simulink model "tether_pull_R2019B"  (R2019b)
settings: Solver=ode4  StartTime=0.0  StopTime=simInit.TSIM  FixedStep=simInit.dt  RelTol=1e-1
InitFcn:
  | close all
undefined symbols (not defined in the file or in its folder): DE2019, ENVMT, simInit, T
libraries: simulink x1, dspmathops x1, dspsigops x1
settings Model: SimulationMode=accelerator  ExtModeTrigDuration=100  Creator=Sebastian  LastModifiedBy=dylaneijkelhof
settings SolverCC: SolverJacobianMethodControl=FullAnalytical
settings DataIOCC: SaveFormat=Array  SaveOutput=off  SignalLogging=off  DSMLogging=off  SaveTime=off  ReturnWorkspaceOutputs=off  StateSaveName=tmp_raccel_xout  SignalLoggingName=logged_signals  LoggingFileName=log
settings OptimizationCC: EfficientMapNaN2IntZero=off
settings DebuggingCC: ArtificialAlgebraicLoopMsg=none  SaveWithDisabledLinksMsg=none  SaveWithParameterizedLinksMsg=none  MaskedZcDiagnostic=none  IgnoredZcDiagnostic=none  InheritedTsInSrcMsg=none  TasksWithSamePriorityMsg=none  SigSpecEnsureSampleTimeMsg=none  ParameterPrecisionLossMsg=none  UnconnectedInputMsg=none  UnconnectedOutputMsg=none  UnconnectedLineMsg=none  BusObjectLabelMismatch=none  RootOutportRequireBusObject=none  AllowSymbolicDim=off  UnknownTsInhSupMsg=none  ModelReferenceDataLoggingMessage=none  ModelReferenceSymbolNameMessage=none  InitInArrayFormatMsg=none  SFUnusedDataAndEventsDiag=none  SFUnexpectedBacktrackingDiag=none  SFInvalidInputDataAccessInChartInitDiag=none  SFNoUnconditionalDefaultTransitionDiag=none  SFTransitionOutsideNaturalParentDiag=none  SFUnreachableExecutionPathDiag=none  SFUndirectedBroadcastEventsDiag=none  SFTransitionActionBeforeConditionDiag=none  SFTemporalDelaySmallerThanSampleTimeDiag=none  SFSelfTransitionDiag=none  SFExecutionAtInitializationDiag=none  SFMachineParentedDataDiag=none  UnitsInconsistencyMsg=none  ArithmeticOperatorsInVariantConditions=warning
settings HardwareCC: ProdBitPerLong=64  ProdHWDeviceType=Intel->x86-64 (Mac OS X)  TargetBitPerLong=64  TargetBitPerPointer=64  TargetBitPerSizeT=64  TargetBitPerPtrDiffT=64  TargetLongLongMode=on  TargetIntDivRoundTo=Zero  TargetEndianess=LittleEndian  TargetWordSize=64  TargetHWDeviceType=MATLAB Host  ProdEqTarget=off
settings ModelReferenceCC: PropagateSignalLabelsOutOfModel=off
settings SFSimCC: SimUseLocalCustomCode=off  CustomCodeUndefinedFunction=UseInterfaceOnly
settings RTWCC: SystemTargetFile=accel.tlc  TemplateMakefile=accel_default_tmf  RTWVerbose=off
settings CodeAppCC: MaxIdLength=128
settings STFCustomTargetCC: TargetLangStandard=C99 (ISO)  ConcurrentExecutionCompliant=on  MATLABClassNameForMDSCustomization=Simulink.SoftwareTarget.TargetSpecificTriggerConfigurationBase  GRTInterface=on  SystemTargetFile=accel.tlc
settings ConfigComp: CovMetricSettings=dw  CovHtmlReporting=on  CovSaveCumulativeToWorkspaceVar=on  CovSaveSingleToWorkspaceVar=on  CovExternalEMLEnable=off

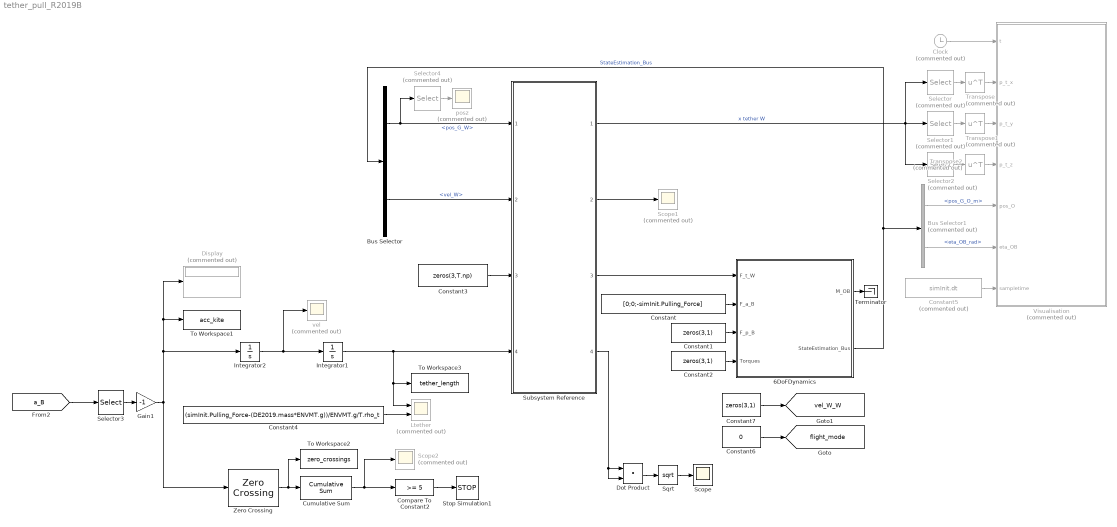
== system tether_pull_R2019B ==
  6DoFDynamics : Subsystem
  Bus Selector : BusSelector  OutputSignals=pos_G_W,vel_W
  Bus Selector1 : BusSelector  Commented=on  OutputSignals=pos_G_O_m,eta_OB_rad
  Clock : Clock  Commented=on
  Compare To Constant2 : simulink/Logic and Bit Operations/Compare To Constant  relop=>=  const=5  OutDataTypeStr=boolean
  Constant : Constant  Value=[0;0;-simInit.Pulling_Force]
  Constant1 : Constant  Value=zeros(3,1)
  Constant2 : Constant  Value=zeros(3,1)
  Constant3 : Constant  Value=zeros(3,T.np)
  Constant4 : Constant  Value=(simInit.Pulling_Force-(DE2019.mass*ENVMT.g))/ENVMT.g/T.rho_t
  Constant5 : Constant  Commented=on  Value=simInit.dt
  Constant6 : Constant  Value=0
  Constant7 : Constant  Value=zeros(3,1)
  Cumulative Sum : dspmathops/Cumulative Sum  dim=Channels (running sum)  InputProcessing=Columns as channels (frame based)  reset_popup=None  roundingMode=Floor  overflowMode=off  outputDataTypeStr=Inherit: Same as accumulator  outputMin=[]  outputMax=[]  outputLastDataTypeStr=Inherit: Same as accumulator
  Display : Display  Commented=on
  Dot Product : DotProduct  InputSameDT=on  OutDataTypeStr=Inherit: Inherit via internal rule
  Gain1 : Gain  Gain=-1
  Integrator1 : Integrator  InitialCondition=T.tether_inital_lenght
  Integrator2 : Integrator
  Ltether : Scope  Commented=on  NumInputPorts=2
  Scope : Scope
  Scope1 : Scope  Commented=on
  Scope2 : Scope  Commented=on
  Selector : Selector  Commented=on  NumberOfDimensions=2  InputPortWidth=3  IndexOptions=Index vector (dialog),Select all  Indices=1,1  OutputSizes=1,1
  Selector1 : Selector  Commented=on  NumberOfDimensions=2  InputPortWidth=3  IndexOptions=Index vector (dialog),Select all  Indices=2,1  OutputSizes=1,1
  Selector2 : Selector  Commented=on  NumberOfDimensions=2  InputPortWidth=3  IndexOptions=Index vector (dialog),Select all  Indices=3,1  OutputSizes=1,1
  Selector3 : Selector  InputPortWidth=3  IndexOptions=Index vector (dialog)  Indices=3  OutputSizes=1
  Selector4 : Selector  Commented=on  InputPortWidth=3  IndexOptions=Index vector (dialog)  Indices=3  OutputSizes=1
  Sqrt : Sqrt  SaturateOnIntegerOverflow=on
  Stop Simulation1 : Stop
  Subsystem Reference : Subsystem  ReferencedSubsystem=Tether_dynamics_R2019B
  Terminator : Terminator
  To Workspace1 : ToWorkspace  VariableName=acc_kite  SaveFormat=Timeseries  SampleTime=-1
  To Workspace2 : ToWorkspace  VariableName=zero_crossings  SaveFormat=Timeseries  SampleTime=-1
  To Workspace3 : ToWorkspace  VariableName=tether_length  SaveFormat=Timeseries  SampleTime=-1
  Transpose : Math  Commented=on  Operator=transpose  SignedPower=off  SaturateOnIntegerOverflow=on
  Transpose1 : Math  Commented=on  Operator=transpose  SignedPower=off  SaturateOnIntegerOverflow=on
  Transpose2 : Math  Commented=on  Operator=transpose  SignedPower=off  SaturateOnIntegerOverflow=on
  Visualisation : MATLAB Function  Commented=on  TreatAsAtomicUnit=on
  Zero Crossing : dspsigops/Zero Crossing  InputProcessing=Columns as channels (frame based)
      settings: SourceProductBaseCode=DS
  posz : Scope  Commented=on
  vel : Scope  Commented=on
  tag scope: flight_mode=global, vel_W_W=global
  wires:
  Subsystem Reference/1 -> Selector2/1, Selector/1, Selector1/1  "x tether W"
  Integrator2/1 -> vel/1, Integrator1/1
  Transpose/1 -> Visualisation/2(p_t_x)
  Integrator1/1 -> Ltether/1, To Workspace3/1, Subsystem Reference/4
  6DoFDynamics/2(StateEstimation_Bus) -> Bus Selector1/1, Bus Selector/1  "StateEstimation_Bus"
  Compare To Constant2/1 -> Stop Simulation1/1
  Constant1/1 -> 6DoFDynamics/3(F_p_B)
  Selector1/1 -> Transpose1/1
  Subsystem Reference/3 -> 6DoFDynamics/1(F_t_W)
  6DoFDynamics/1(M_OB) -> Terminator/1
  Constant2/1 -> 6DoFDynamics/4(Torques)
  Bus Selector/1 -> Subsystem Reference/1, Selector4/1  "<pos_G_W>"
  Subsystem Reference/2 -> Scope1/1
  Bus Selector/2 -> Subsystem Reference/2  "<vel_W>"
  Constant/1 -> 6DoFDynamics/2(F_a_B)
  Clock/1 -> Visualisation/1(t)
  Selector2/1 -> Transpose2/1
  Selector/1 -> Transpose/1
  Constant5/1 -> Visualisation/7(sampletime)
  Constant3/1 -> Subsystem Reference/3
  Transpose1/1 -> Visualisation/3(p_t_y)
  Bus Selector1/2 -> Visualisation/6(eta_OB)  "<eta_OB_rad>"
  Transpose2/1 -> Visualisation/4(p_t_z)
  Bus Selector1/1 -> Visualisation/5(pos_O)  "<pos_G_O_m>"
  Selector4/1 -> posz/1
  Constant4/1 -> Ltether/2
  [a_B] -> Selector3/1
  Selector3/1 -> Gain1/1
  Zero Crossing/1 -> To Workspace2/1, Cumulative Sum/1
  Cumulative Sum/1 -> Scope2/1, Compare To Constant2/1
  Gain1/1 -> Display/1, To Workspace1/1, Integrator2/1, Zero Crossing/1
  Constant6/1 -> [flight_mode]
  Constant7/1 -> [vel_W_W]
  Subsystem Reference/4 -> Dot Product/2, Dot Product/1
  Dot Product/1 -> Sqrt/1
  Sqrt/1 -> Scope/1

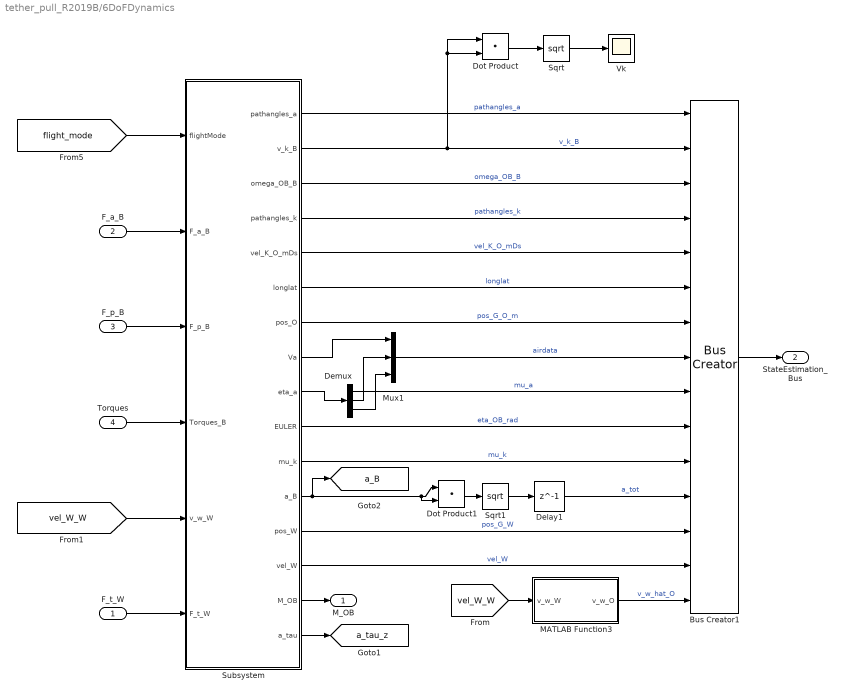
== system tether_pull_R2019B/6DoFDynamics ==
  F_t_W : Inport
  F_a_B : Inport  Port=2
  F_p_B : Inport  Port=3
  Torques : Inport  Port=4
  Bus Creator1 : BusCreator  Inputs=15
  Delay1 : Delay  DelayLength=1
  Demux : Demux  Outputs=3
  Dot Product : DotProduct  InputSameDT=on  OutDataTypeStr=Inherit: Inherit via internal rule
  Dot Product1 : DotProduct  InputSameDT=on  OutDataTypeStr=Inherit: Inherit via internal rule
  MATLAB Function3 : MATLAB Function  TreatAsAtomicUnit=on
  Mux1 : Mux  Inputs=3
  Sqrt : Sqrt  SaturateOnIntegerOverflow=on
  Sqrt1 : Sqrt  SaturateOnIntegerOverflow=on
  Subsystem : Subsystem
  Vk : Scope
  M_OB : Outport  PortDimensions=[3,3]  VectorParamsAs1DForOutWhenUnconnected=off
  StateEstimation_Bus : Outport  Port=2  VectorParamsAs1DForOutWhenUnconnected=off
  tag scope: a_B=global, a_tau_z=global
  wires:
  Demux/1 -> Bus Creator1/9  "mu_a"
  Subsystem/15(M_OB) -> M_OB/1
  Subsystem/8(Va) -> Mux1/1
  Subsystem/1(pathangles_a) -> Bus Creator1/1  "pathangles_a"
  [vel_W_W] -> Subsystem/5(v_w_W)
  Torques/1 -> Subsystem/4(Torques_B)
  F_p_B/1 -> Subsystem/3(F_p_B)
  F_a_B/1 -> Subsystem/2(F_a_B)
  [flight_mode] -> Subsystem/1(flightMode)
  Subsystem/4(pathangles_k) -> Bus Creator1/4  "pathangles_k"
  Subsystem/2(v_k_B) -> Bus Creator1/2, Dot Product/1, Dot Product/2  "v_k_B"
  Subsystem/10(EULER) -> Bus Creator1/10  "eta_OB_rad"
  Subsystem/6(longlat) -> Bus Creator1/6  "longlat"
  Subsystem/5(vel_K_O_mDs) -> Bus Creator1/5  "vel_K_O_mDs"
  Bus Creator1/1 -> StateEstimation_Bus/1
  Subsystem/3(omega_OB_B) -> Bus Creator1/3  "omega_OB_B"
  Subsystem/7(pos_O) -> Bus Creator1/7  "pos_G_O_m"
  Demux/3 -> Mux1/3
  Subsystem/9(eta_a) -> Demux/1
  Delay1/1 -> Bus Creator1/12  "a_tot"
  Sqrt1/1 -> Delay1/1
  Dot Product1/1 -> Sqrt1/1
  Subsystem/12(a_B) -> Dot Product1/1, Dot Product1/2, [a_B]
  Subsystem/11(mu_k) -> Bus Creator1/11  "mu_k"
  MATLAB Function3/1(v_w_O) -> Bus Creator1/15  "v_w_hat_O"
  [vel_W_W] -> MATLAB Function3/1(v_w_W)
  Mux1/1 -> Bus Creator1/8  "airdata"
  Demux/2 -> Mux1/2
  F_t_W/1 -> Subsystem/6(F_t_W)
  Subsystem/13(pos_W) -> Bus Creator1/13  "pos_G_W"
  Subsystem/14(vel_W) -> Bus Creator1/14  "vel_W"
  Subsystem/16(a_tau) -> [a_tau_z]
  Sqrt/1 -> Vk/1
  Dot Product/1 -> Sqrt/1

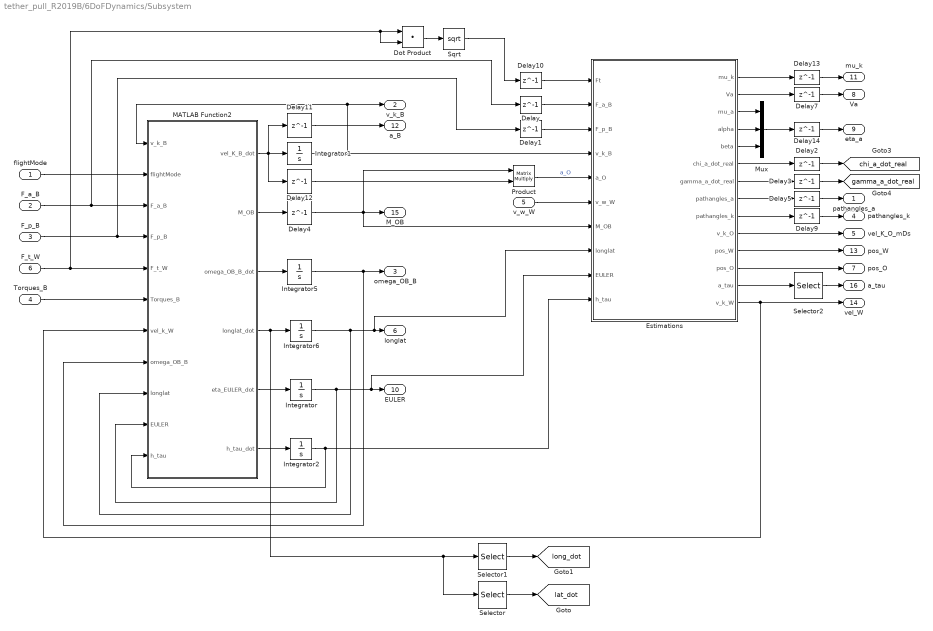
== system tether_pull_R2019B/6DoFDynamics/Subsystem ==
  flightMode : Inport
  F_a_B : Inport  Port=2  PortDimensions=[3,1]
  F_p_B : Inport  Port=3
  Torques_B : Inport  Port=4  PortDimensions=[3,1]
  v_w_W : Inport  Port=5  PortDimensions=[3,1]
  F_t_W : Inport  Port=6
  Delay{,1,11..12,14} (5 alike) : Delay  DelayLength=1  InitialCondition=zeros(3,1)
  Delay10 : Delay  DelayLength=1  InitialCondition=0
  Delay13 : Delay  DelayLength=1  InitialCondition=0
  Delay2 : Delay  DelayLength=1
  Delay3 : Delay  DelayLength=1
  Delay4 : Delay  DelayLength=1  InitialCondition=eye(3)
  Delay5 : Delay  DelayLength=1  InitialCondition=zeros(2,1)
  Delay7 : Delay  DelayLength=1  InitialCondition=simInit.vel_B_init(1)
  Delay9 : Delay  DelayLength=1  InitialCondition=zeros(2,1)
  Dot Product : DotProduct  InputSameDT=on  OutDataTypeStr=Inherit: Inherit via internal rule
  Estimations : MATLAB Function  TreatAsAtomicUnit=on
  Integrator : Integrator  InitialCondition=simInit.eta_init  WrapState=on
  Integrator1 : Integrator  InitialCondition=simInit.vel_B_init
  Integrator2 : Integrator  InitialCondition=norm(simInit.pos_O_init)
  Integrator5 : Integrator  InitialCondition=zeros(3,1)
  Integrator6 : Integrator  InitialCondition=[simInit.long_init;simInit.lat_init]  WrapState=on
  MATLAB Function2 : MATLAB Function  TreatAsAtomicUnit=on
  Mux : Mux  Inputs=3
  Product : Product  Multiplication=Matrix(*)
  Selector : Selector  InputPortWidth=2  IndexOptions=Index vector (dialog)  Indices=2  OutputSizes=1
  Selector1 : Selector  InputPortWidth=2  IndexOptions=Index vector (dialog)  Indices=1  OutputSizes=1
  Selector2 : Selector  InputPortWidth=3  IndexOptions=Index vector (dialog)  Indices=3  OutputSizes=1
  Sqrt : Sqrt  SaturateOnIntegerOverflow=on
  pathangles_a : Outport  PortDimensions=[2,1]  VectorParamsAs1DForOutWhenUnconnected=off
  v_k_B : Outport  Port=2  PortDimensions=[3,1]  VectorParamsAs1DForOutWhenUnconnected=off
  omega_OB_B : Outport  Port=3  PortDimensions=[3,1]  VectorParamsAs1DForOutWhenUnconnected=off
  pathangles_k : Outport  Port=4  PortDimensions=[2,1]  VectorParamsAs1DForOutWhenUnconnected=off
  vel_K_O_mDs : Outport  Port=5  PortDimensions=[3,1]  VectorParamsAs1DForOutWhenUnconnected=off
  longlat : Outport  Port=6  PortDimensions=[2,1]  VectorParamsAs1DForOutWhenUnconnected=off
  pos_O : Outport  Port=7  PortDimensions=[3,1]  VectorParamsAs1DForOutWhenUnconnected=off
  Va : Outport  Port=8  PortDimensions=1  VectorParamsAs1DForOutWhenUnconnected=off
  eta_a : Outport  Port=9  PortDimensions=[3,1]  VectorParamsAs1DForOutWhenUnconnected=off
  EULER : Outport  Port=10  PortDimensions=[3,1]  VectorParamsAs1DForOutWhenUnconnected=off
  mu_k : Outport  Port=11  PortDimensions=1  VectorParamsAs1DForOutWhenUnconnected=off
  a_B : Outport  Port=12  PortDimensions=[3,1]  VectorParamsAs1DForOutWhenUnconnected=off
  pos_W : Outport  Port=13  PortDimensions=[3,1]  VectorParamsAs1DForOutWhenUnconnected=off
  vel_W : Outport  Port=14  PortDimensions=[3,1]  VectorParamsAs1DForOutWhenUnconnected=off
  M_OB : Outport  Port=15  PortDimensions=[3,3]  VectorParamsAs1DForOutWhenUnconnected=off
  a_tau : Outport  Port=16  PortDimensions=1  VectorParamsAs1DForOutWhenUnconnected=off
  tag scope: chi_a_dot_real=global, gamma_a_dot_real=global, lat_dot=global, long_dot=global
  wires:
  Delay5/1 -> pathangles_a/1
  Delay4/1 -> M_OB/1, Product/1, Estimations/7(M_OB)
  Torques_B/1 -> MATLAB Function2/6(Torques_B)
  MATLAB Function2/2(M_OB) -> Delay4/1
  F_a_B/1 -> Delay/1, MATLAB Function2/3(F_a_B)
  Mux/1 -> Delay14/1
  MATLAB Function2/3(omega_OB_B_dot) -> Integrator5/1
  MATLAB Function2/4(longlat_dot) -> Integrator6/1, Selector/1, Selector1/1
  MATLAB Function2/1(vel_K_B_dot) -> Delay12/1, Delay11/1, Integrator1/1
  flightMode/1 -> MATLAB Function2/2(flightMode)
  v_w_W/1 -> Estimations/6(v_w_W)
  Integrator1/1 -> Estimations/4(v_k_B), MATLAB Function2/1(v_k_B), v_k_B/1
  F_p_B/1 -> Delay1/1, MATLAB Function2/4(F_p_B)
  Estimations/8(pathangles_a) -> Delay5/1
  Estimations/9(pathangles_k) -> Delay9/1
  Estimations/2(Va) -> Delay7/1
  Delay7/1 -> Va/1
  Estimations/3(mu_a) -> Mux/1
  Delay2/1 -> [chi_a_dot_real]
  Estimations/6(chi_a_dot_real) -> Delay2/1
  Estimations/7(gamma_a_dot_real) -> Delay3/1
  Delay3/1 -> [gamma_a_dot_real]
  MATLAB Function2/5(eta_EULER_dot) -> Integrator/1
  Integrator/1 -> MATLAB Function2/10(EULER), Estimations/9(EULER), EULER/1
  Integrator5/1 -> MATLAB Function2/8(omega_OB_B), omega_OB_B/1
  Estimations/1(mu_k) -> Delay13/1
  Integrator6/1 -> MATLAB Function2/9(longlat), Estimations/8(longlat), longlat/1
  Delay13/1 -> mu_k/1
  Delay14/1 -> eta_a/1
  Delay9/1 -> pathangles_k/1
  Estimations/4(alpha) -> Mux/2
  Estimations/5(beta) -> Mux/3
  F_t_W/1 -> Dot Product/1, Dot Product/2, MATLAB Function2/5(F_t_W)
  Dot Product/1 -> Sqrt/1
  Sqrt/1 -> Delay10/1
  Delay11/1 -> a_B/1
  MATLAB Function2/6(h_tau_dot) -> Integrator2/1
  Integrator2/1 -> MATLAB Function2/11(h_tau), Estimations/10(h_tau)
  Estimations/12(pos_O) -> pos_O/1
  Estimations/14(v_k_W) -> vel_W/1, MATLAB Function2/7(vel_k_W)
  Estimations/11(pos_W) -> pos_W/1
  Estimations/10(v_k_O) -> vel_K_O_mDs/1
  Delay/1 -> Estimations/2(F_a_B)
  Delay1/1 -> Estimations/3(F_p_B)
  Delay10/1 -> Estimations/1(Ft)
  Selector/1 -> [lat_dot]
  Selector1/1 -> [long_dot]
  Product/1 -> Estimations/5(a_O)  "a_O"
  Estimations/13(a_tau) -> Selector2/1
  Delay12/1 -> Product/2
  Selector2/1 -> a_tau/1

== matlab function tether_pull_R2019B/6DoFDynamics/Subsystem/Estimations ==
  data: Ft input; F_a_B input; F_p_B input; v_k_B input; a_O input; v_w_W input; mu_k output; Va output; mu_a output; alpha output; beta output; chi_a_dot_real output; gamma_a_dot_real output; M_OB input; longlat input; EULER input; pathangles_a output; pathangles_k output; v_k_O output; pos_W output; pos_O output; a_tau output; ENVMT parameter; DE2019 parameter; v_k_W output; h_tau input
function [mu_k,Va, mu_a, alpha, beta, chi_a_dot_real,gamma_a_dot_real, pathangles_a, pathangles_k, v_k_O, pos_W, pos_O,a_tau, v_k_W] = fcn(Ft, F_a_B, F_p_B, v_k_B, a_O, v_w_W,M_OB,longlat,EULER,...
    ENVMT, DE2019, h_tau)

mu_k = 0;
Va = 0;
mu_a = 0;
alpha =0; 
beta=0;
chi_a_dot_real=0;
gamma_a_dot_real=0;
pathangles_a =zeros(2,1);
pathangles_k=zeros(2,1); 
chi_a_dot_real2=0;
gamma_a_dot_real2=0; 

long = longlat(1);
lat = longlat(2);

M_WO = [cos(ENVMT.windDirection_rad), sin(ENVMT.windDirection_rad), 0;
        sin(ENVMT.windDirection_rad), -cos(ENVMT.windDirection_rad), 0;
        0, 0, -1];

 a_W = M_WO*a_O;

phi = longlat(2);
lamb = longlat(1);

M_tauW = [-sin(phi)*cos(lamb), -sin(phi)*sin(lamb), cos(phi);
    -sin(lamb), cos(lamb), 0;
    -cos(phi)*cos(lamb), -cos(phi)*sin(lamb), -sin(phi)];
a_tau = M_tauW*a_W;
%a_tau = zeros(3,1);    
pos_W = [cos(long)*cos(lat);
         sin(long)*cos(lat);
         sin(lat)]*abs(h_tau);
    
pos_O = M_WO'*pos_W;   
v_k_O = M_OB*v_k_B;
v_k_W =  M_WO*v_k_O;

v_a_W = v_k_W - v_w_W;
Va = norm(v_a_W);

v_a_O = transformFromWtoO(ENVMT.windDirection_rad, v_a_W);
v_a_B = M_OB' * v_a_O;

chi_k = atan2( v_k_O(2), v_k_O(1) );
gamma_k = -asin( v_k_O(3)/norm(v_k_O) );
pathangles_k = [chi_k; gamma_k];

chi_a = atan2( v_a_O(2), v_a_O(1) );
gamma_a = -asin( v_a_O(3)/norm(v_a_O) );
pathangles_a = [chi_a; gamma_a];

% Estimation of aerodynamic angles 
alpha = 0;
beta = 0;
mu_a = 0;
alpha = atan2( v_a_B(3), v_a_B(1) );
beta = asin( v_a_B(2)/norm(v_a_B) );
mu_a= asin( max( min( (cos(EULER(2))*sin(EULER(1)))/(cos(gamma_a)*cos(beta)) + tan(gamma_a) * tan(beta), 1),-1) ); 

beta_k = atan2( v_k_B(2), norm(v_k_B) );
mu_k = 0;
mu_k= asin( max( min( (cos(EULER(2))*sin(EULER(1)))/(cos(gamma_k)*cos(beta_k)) + tan(gamma_k) * tan(beta_k), 1),-1) ); 

c_m = cos(mu_a);
s_m = sin(mu_a);

c_a = cos(alpha);
s_a = sin(alpha);

c_b = cos(beta);
s_b = sin(beta);

M_B2ABar = zeros(3,3);

M_B2ABar(1,1) = c_a*c_b;
M_B2ABar(1,2) = s_b;
M_B2ABar(1,3) = s_a*c_b;
M_B2ABar(2,1) = -c_a*s_b*c_m+s_a*s_m;
M_B2ABar(2,2) = c_b*c_m;
M_B2ABar(2,3) = -s_a*s_b*c_m-s_m*c_a;
M_B2ABar(3,1) = -c_a*s_b*s_m-s_a*c_m;
M_B2ABar(3,2) = c_b*s_m;
M_B2ABar(3,3) = -s_a*s_b*s_m+c_a*c_m;

% Estimtion of chi_a_dot and gamma_a_dot

c_chia = cos(chi_a);
s_chia = sin(chi_a);

c_gama = cos(gamma_a);
s_gama = sin(gamma_a);

M_ABar2O = zeros(3,3);

M_ABar2O(1,1) = c_chia*c_gama;
M_ABar2O(2,1) = s_chia*c_gama;
M_ABar2O(3,1) = -s_gama;
M_ABar2O(1,2) = -s_chia;
M_ABar2O(2,2) = c_chia;
M_ABar2O(3,2) = 0;
M_ABar2O(1,3) = c_chia*s_gama;
M_ABar2O(2,3) = s_chia*s_gama;
M_ABar2O(3,3) = c_gama;


F_g_t_Abar = M_ABar2O' * ( [0;0;DE2019.mass*ENVMT.g] -Ft*pos_O/norm(pos_O) );
F_ap_B = M_B2ABar * (F_a_B+F_p_B);
f_y = F_ap_B(2) + F_g_t_Abar(2); 
f_z = F_ap_B(3) + F_g_t_Abar(3);

chi_a_dot_real = 0;
gamma_a_dot_real = 0;
chi_a_dot_real = 1/cos(gamma_a)/Va/DE2019.mass  * (f_y);
gamma_a_dot_real = -1/Va/DE2019.mass * (f_z);

chi_a_dot_real2 = 0;
gamma_a_dot_real2 = 0;

% this does not work perfectly because of the wind.
% chi_a_dot_real2 = 1/cos(gamma_a)/Va *a_Abar(2);
% gamma_a_dot_real2 = -1/Va*(a_Abar(3)+cos(gamma_a)*ENVMT.g);

end

== matlab function tether_pull_R2019B/6DoFDynamics/Subsystem/MATLAB Function2 ==
  data: v_k_B input; flightMode input; DE2019 parameter; F_a_B input; F_p_B input; ENVMT parameter; F_t_W input; Torques_B input; vel_k_W input; omega_OB_B input; longlat input; EULER input; h_tau input; vel_K_B_dot output; M_OB output; omega_OB_B_dot output; longlat_dot output; eta_EULER_dot output; h_tau_dot output
function [vel_K_B_dot, M_OB, omega_OB_B_dot, longlat_dot, eta_EULER_dot, h_tau_dot] = fcn(v_k_B, flightMode, DE2019, F_a_B, F_p_B ,...
    ENVMT, F_t_W, Torques_B, vel_k_W, omega_OB_B, longlat, EULER, h_tau)

x_tau_2dot = 0;
y_tau_2dot = 0;
z_tau_2dot = 0;
z_tau_2dot_unsat = 0;

omega_OB_B_dot = zeros(3,1);
eta_EULER_dot = zeros(3,1);
longlat_dot = zeros(2,1);
vel_K_B_dot = zeros(3,1);

c_psi = cos(EULER(3));
s_psi = sin(EULER(3));

c_theta = cos(EULER(2));
s_theta = sin(EULER(2));

c_phi = cos(EULER(1));
s_phi = sin(EULER(1)); 

M_OB = [ c_psi*c_theta, c_psi*s_theta*s_phi-s_psi*c_phi, c_psi*s_theta*c_phi+s_psi*s_phi;
         s_psi*c_theta, s_psi*s_theta*s_phi+c_psi*c_phi, s_psi*s_theta*c_phi-c_psi*s_phi;
        -s_theta, c_theta*s_phi, c_theta*c_phi];

long = longlat(1);
lat = longlat(2);

F_g_O = [0;0;DE2019.mass*ENVMT.g];
F_t_O = transformFromOtoW( ENVMT.windDirection_rad, F_t_W);

if flightMode == 2
    Forces_B = F_a_B +  M_OB'*F_g_O + F_p_B;
else
    F_g_B = M_OB'*(F_g_O+F_t_O);
    Forces_B = F_a_B + F_g_B + F_p_B ;
end


p=omega_OB_B(1);
q=omega_OB_B(2);
r=omega_OB_B(3);

u=v_k_B(1);
v=v_k_B(2);
w=v_k_B(3);
vel_K_B_dot = [r*v-q*w + 1/DE2019.mass * Forces_B(1);
               p*w-r*u + 1/DE2019.mass * Forces_B(2);
               q*u-p*v + 1/DE2019.mass * Forces_B(3)];

c_theta = cos(EULER(2));
s_theta = sin(EULER(2));

c_phi = cos(EULER(1));
s_phi = sin(EULER(1)); 

eta_EULER_dot = [1 s_phi*s_theta/c_theta c_phi*s_theta/c_theta;
                 0 c_phi -s_phi; 
                 0 s_phi/c_theta c_phi/c_theta]*omega_OB_B;

Gamma = DE2019.Jx*DE2019.Jz-DE2019.Jxz^2;
Gamma1 = (DE2019.Jxz*(DE2019.Jx - DE2019.Jy + DE2019.Jz ))/Gamma;
Gamma2 = (DE2019.Jz * (DE2019.Jz - DE2019.Jy) + DE2019.Jxz^2)/Gamma;
Gamma3 = DE2019.Jz/Gamma;
Gamma4 = DE2019.Jxz/Gamma;
Gamma5 = (DE2019.Jz - DE2019.Jx)/DE2019.Jy;
Gamma6 = DE2019.Jxz / DE2019.Jy;
Gamma7 = ((DE2019.Jx - DE2019.Jy)*DE2019.Jx + DE2019.Jxz^2 )/Gamma;
Gamma8 = DE2019.Jx / Gamma;

omega_OB_B_dot = [Gamma1 * p * q - Gamma2 * q * r + Gamma3 * Torques_B(1) + Gamma4 * Torques_B(3);
    Gamma5 * p * r - Gamma6 * (p^2 - r^2) + 1/DE2019.Jy *Torques_B(2);
     Gamma7 * p * q - Gamma1 * q * r + Gamma4 * Torques_B(1) + Gamma8 * Torques_B(3)];

%% Position propagation
sin_lat = sin(lat);
sin_long =sin(long);
cos_lat = cos(lat);
cos_long = cos(long);
 
M_tauW = [-sin_lat*cos_long, -sin_lat*sin_long,cos_lat;
    -sin_long, cos_long, 0;
    -cos_lat*cos_long, -cos_lat*sin_long, -sin_lat];

v_k_tau =M_tauW*vel_k_W;

long_dot = v_k_tau(2)/( abs(h_tau)*cos(lat));
lat_dot = v_k_tau(1)/abs(h_tau);

h_tau_dot = -v_k_tau(3);

longlat_dot = [long_dot;
               lat_dot];


end

== matlab function tether_pull_R2019B/Visualisation ==
  settings: updateMethod=DISCRETE
  data: t input; p_t_x input; p_t_y input; p_t_z input; pos_O input; eta_OB input; ENVMT parameter; sampletime input
function Visualisation(t,p_t_x,p_t_y,p_t_z, pos_O,eta_OB, ENVMT, sampletime)   
    persistent handleTether
    persistent Vert
    persistent handlePlane
    
    coder.extrinsic('plot3','patch');
 
    %% Figure settings
    if t==0
        figure(99)
%         addToolbarExplorationButtons(gcf)
        xlabel('x_W (m)');%, 'interpreter', 'latex')
        ylabel('y_W (m)');%, 'interpreter', 'latex')
        zlabel('z_W (m)');%, 'interpreter', 'latex')

        grid on
        box on;
        axis equal; hold on;

        view(30,21); % set the vieew angle for figure

        ax = [-500 1500];
        ay = [-600 600];
        az = [0 1200];
        axis([ax,ay,az]);  hold on

        X = [ax(1);ax(2);ax(2);ax(1)];
        Y = [ay(1);ay(1);ay(2);ay(2)];
        Z = [0;0;0;0];

        c = [0 1 0; % red
        0 1 0; % green
        0 1 0;
        0 1 0];
        fill3(X,Y,Z, c(:,2),'EdgeColor','none','FaceColor',c(1,:),'FaceAlpha',0.1);
    end
    
    %% Draw tether particles
    if isempty(handleTether)
 
        M_WO = [cos(ENVMT.windDirection_rad), sin(ENVMT.windDirection_rad), 0;
        sin(ENVMT.windDirection_rad), -cos(ENVMT.windDirection_rad), 0;
        0, 0, -1];
        pos_W = M_WO*[pos_O(1);pos_O(2);pos_O(3)];
        handleTether = plot3( [0;p_t_x;pos_W(1)], [0;p_t_y;pos_W(2)],[0;p_t_z;pos_W(3)],...
            '-', 'color', [0.1 0.1 0.1], 'Markersize',2, 'Linewidth', 1.2,...
            'MarkerFaceColor', [0.3 0.3 0.3]); hold on;
    end
    
    %% Draw aircraft
    if isempty(handlePlane)
        pn = pos_O(1);
        pe = pos_O(2);
        pd = pos_O(3);
        phi = eta_OB(1);
        theta = eta_OB(2);
        psi = eta_OB(3);
        
        M_WO = [cos(ENVMT.windDirection_rad), sin(ENVMT.windDirection_rad), 0;
        sin(ENVMT.windDirection_rad), -cos(ENVMT.windDirection_rad), 0;
        0, 0, -1];
        
        scale = 6;
%         [F, Vert, C] = rndread('plane_thesis_big.stl');
        Image_kite = coder.load('plane_image.mat','F','Verti','C');
        F = Image_kite.F;
        Verti = Image_kite.Verti;
        C = Image_kite.C;
        Vert = scale*Verti'; 
        V = [ cos(psi)*cos(theta) , cos(psi)*sin(phi)*sin(theta) - cos(phi)*sin(psi) , sin(phi)*sin(psi) + cos(phi)*cos(psi)*sin(theta);
            cos(theta)*sin(psi)   , cos(phi)*cos(psi) + sin(phi)*sin(psi)*sin(theta) , cos(phi)*sin(psi)*sin(theta) - cos(psi)*sin(phi);
               -sin(theta)        ,             cos(theta)*sin(phi)                  ,             cos(phi)*cos(theta)                 ]...
               * Vert;
        V = V + [pn*ones(1,size(V,2));pe*ones(1,size(V,2));pd*ones(1,size(V,2))];
        V = M_WO*V;
        col =  [ 57/255, 106/255, 177/255  ];
        handlePlane = patch('faces', F, 'vertices' ,V');
        set(handlePlane, 'facec', 'b');              % Set the face color (force it)
        set(handlePlane, 'FaceVertexCData', C);       % Set the color (from file)
        set(handlePlane, 'EdgeColor','none');
        set(handlePlane, 'FaceLighting', 'none');
        set(handlePlane, 'FaceColor', col );
    end
    
    if (mod(t,sampletime)==0 && t~=0)
        %% Change each element on figure to current positions
        
        pn = pos_O(1);
        pe = pos_O(2);
        pd = pos_O(3);
        phi = eta_OB(1);
        theta = eta_OB(2);
        psi = eta_OB(3);
        
        M_WO = [cos(ENVMT.windDirection_rad), sin(ENVMT.windDirection_rad), 0;
        sin(ENVMT.windDirection_rad), -cos(ENVMT.windDirection_rad), 0;
        0, 0, -1];
        
        % Tether
        set(handleTether,'XData',[0;p_t_x;-pn], 'YData',[0;p_t_y;pe],'ZData',[0;p_t_z;-pd]);
        
        % Kite
        V = [ cos(psi)*cos(theta), cos(psi)*sin(phi)*sin(theta) - cos(phi)*sin(psi), sin(phi)*sin(psi) + cos(phi)*cos(psi)*sin(theta);
            cos(theta)*sin(psi), cos(phi)*cos(psi) + sin(phi)*sin(psi)*sin(theta), cos(phi)*sin(psi)*sin(theta) - cos(psi)*sin(phi);
            -sin(theta),                              cos(theta)*sin(phi),                              cos(phi)*cos(theta)] * Vert;
        V = V + [pn*ones(1,size(V,2));pe*ones(1,size(V,2));pd*ones(1,size(V,2))];
        V = M_WO*V;
        set(handlePlane, 'Vertices', V');  
        
    end

== matlab function tether_pull_R2019B/6DoFDynamics/MATLAB Function3 ==
  data: v_w_O output; v_w_W input; ENVMT parameter
function v_w_O = fcn(v_w_W, ENVMT)

v_w_O = transformFromWtoO(ENVMT.windDirection_rad, v_w_W );
